simulink library "RTXeno_DataAcquisitionlib"  (Simulink 7.8)
settings: Solver=ode45  StartTime=0.0  StopTime=10.0  RelTol=1e-3
settings Model: Creator=root  LastModifiedBy=root

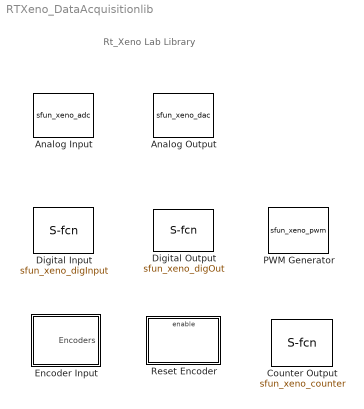
== system RTXeno_DataAcquisitionlib ==
  note: Rt_Xeno Lab Library
  Analog Input : S-Function  FunctionName=sfun_xeno_adc  Parameters=channel,range  EnableBusSupport=off  mask(RTXeno-Lab A/D Converter Block ){channel=[ 0 1 2 3 4 5 6 7], range=0}
      mask prompts: channel "Analog Input Channels"; range "Operation Range"
      mask help:
      | This block is used to select A/D converter parameters for selected data acquisition device.
      | Parameters are analog input channel(s) to use, operation mode. Operation mode is a scalar entry.
      | Other parameter is an array whose size must be same as number of analog input channels, e.g [0 1 ..]
      mask Display: fprintf('ADC')
  Analog Output : S-Function  Tag=sss  FunctionName=sfun_xeno_dac  Parameters=channel,mode,val,fval  EnableBusSupport=off  mask(RTXeno-Lab D/A Converter Block ){channel=[0 0 0 0 0 0 0 0], mode=Bipolar 10V, val=[0 0 0 0 0 0 0 0], fval=[0 0 0 0 0 0 0 0]}
      mask prompts: channel "Analog Output Channel(s)"; mode "Operation Mode"; val "Initial Value(s)"; fval "Final Value(s)"
      mask help:
      | This block is used to select D/A converter parameters for selected data acquisition device.
      | Parameters are analog output channel(s), operation mode, initial value(s) and final value(s). Operation mode is a scalar entry.
      | Other parameters are arrays whose size must be same as number of analog output channels, e.g [0 1 ..]
      mask StyleString: edit,popup(Unipolar 10V|Bipolar 5V|Bipolar 10V),edit,edit
      mask Display: fprintf('DAC');
  Counter Output : S-Function  FunctionName=sfun_xeno_counter  Parameters=clock,period,cntrlen  EnableBusSupport=off  mask(RTXenoLab Counter Block){clock=Counter, period=0, cntrlen=0}
      mask prompts: clock "Clock Source"
      mask help:
      | Counter block produces square wave signal based on user defined period.
      | Also, clock source can be selected according to the hardware.
      mask StyleString: popup(Counter|Watchdog),edit,edit
      mask Display: fprintf('Counter');
  Digital Input : S-Function  FunctionName=sfun_xeno_digInput  Parameters=channels  EnableBusSupport=off  mask(RTXenoLab Digital Input Block){channels=[0]}
      mask prompts: channels "Digita Input Channel(s)"
      mask help:
      | This block is used to configure digital output device for selected data acquisition device.
      | Parameters are digital input channel(s) to use.
      |     All parameters must be entered as array elements. For example  For example if the user wants to use channel 4 then he/she must edit related parameter area  [4].
      mask Display: fprintf(' Digital\nInput');
  Digital Output : S-Function  FunctionName=sfun_xeno_digOut  Parameters=channels,initVal,finalVal  EnableBusSupport=off  mask(RTXenoLab Digital Output Block){channels=[0 1 2 3 4 5 6 7], initVal=[0 0 0 0 0 0 0 0], finalVal=[0 0 0 0 0 0 0 0]}
      mask prompts: channels "Digital Output Channel(s)"; initVal "Initial Value(s)"; finalVal "Final Value(s)"
      mask help:
      | This block is used to configure digital output device for selected data acquisition device.
      | Parameters are digital output channel(s) to use,initial value(s),final value(s).
      |     All parameters must be entered as array elements. For example if the user wants to use channel 4 then he/she must edit related parameter area  [4].
      mask Help:
      | Edit digital output channel(s) parameter as [0 ...31...],
      | Edit digital initial and final value(s) as [0...1 1 1....] etc.
      mask Display: fprintf(' Digital\n Output');
  Encoder Input : Subsystem  mask(RTXenoLab Encoder Input Block){channel=[0 1], cmode=Normal, bmode=Binary, qmode=1X, index=on, indexpole=Positive, reset=on, set=[0 0]}
      mask prompts: channel "Encoder Channel(s)"; cmode "Count Mode"; bmode "Binary/Bcd Mode"; qmode "Quadrature Mode"; index "Index Enable"; indexpole "Index Polarity"; reset "Reset Encoder"; set "Offset"
      mask help: This block is used to configure and read multiple encoder pulses from data acquisition devices.
      mask StyleString: edit,popup(Normal|Range Limit|Non-Recycle|Modulo-N),popup(Binary|BCD),popup(1X|2X|3X|4X),checkbox,popup(Positive|Negative),checkbox,edit
      mask Display: fprintf('Encoder');
  PWM Generator : S-Function  FunctionName=sfun_xeno_pwm  Parameters=clock,period,cntrlen  EnableBusSupport=off  mask(RTXenoLab PWM Generator){clock=WatchDog, period=0.5, cntrlen=on}
      mask prompts: clock "Clock Source"
      mask help:
      | PWM generator produces pwm signal based on user defined period and pulse width.
      | Also, clock source can be selected according to the hardware.
      mask StyleString: popup(Counter|WatchDog),edit,checkbox
      mask Display: fprintf('PWM');
  Reset Encoder : Subsystem  mask{channel=[0 1], cmode=Normal, bmode=Binary, qmode=1X, index=on, indexpole=Positive, reset=on, set=[0 0 ]}
      mask prompts: channel "Encoder Channel(s)"; cmode "Count Mode"; bmode "Binary/Bcd Mode"; qmode "Quadrature Mode"; index "Index Enable"; indexpole "Index Polarity"; reset "Reset Encoder"; set "Offset"
      mask StyleString: edit,popup(Normal|Range Limit|Non-Recycle|Modulo-N),popup(Binary|Bcd),popup(1X|2X|3X|4X),checkbox,popup(Positive|Negative),checkbox,edit

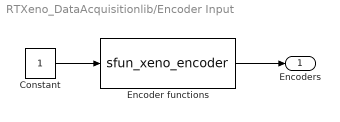
== system RTXeno_DataAcquisitionlib/Encoder Input ==
  Constant : Constant
  Encoder functions : S-Function  FunctionName=sfun_xeno_encoder  Parameters=channel,cmode,bmode,qmode,index,indexpole,reset,set  EnableBusSupport=off
  Encoders : Outport
  wires:
  Constant/1 -> Encoder functions/1
  Encoder functions/1 -> Encoders/1

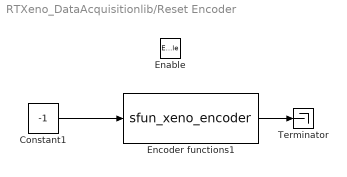
== system RTXeno_DataAcquisitionlib/Reset Encoder ==
  Enable : EnablePort
  Constant1 : Constant  Value=-1
  Encoder functions1 : S-Function  FunctionName=sfun_xeno_encoder  Parameters=channel,cmode,bmode,qmode,index,indexpole,reset,set  EnableBusSupport=off
  Terminator : Terminator
  wires:
  Constant1/1 -> Encoder functions1/1
  Encoder functions1/1 -> Terminator/1
